simulink model "adip_least_square_MN_sim"  (R2013a)
settings: Solver=ode1  StartTime=0.0  StopTime=max(t)  FixedStep=0.001  RelTol=1e-3
values from neighbouring files (symbols this model uses):
  alpha3 = m2*L1*l2    (= 0.00424944)    [p1c332_adip_id_least_square.m]
  alpha5 = m2*l2*g    (= 0.1836432)    [p1c332_adip_id_least_square.m]
  Tf1 = 0.075    [p1c322_cdip_id_least_square.m]    (also in p1c322_cdip_plot_MN.m = 0.05; p1c332_adip_id_least_square.m)
  Tf2 = 0.075    [p1c322_cdip_id_least_square.m]    (also in p1c322_cdip_plot_MN.m = 0.05; p1c332_adip_id_least_square.m)
libraries: cstblocks x6
settings Model: Creator=kawata  LastModifiedBy=kawata

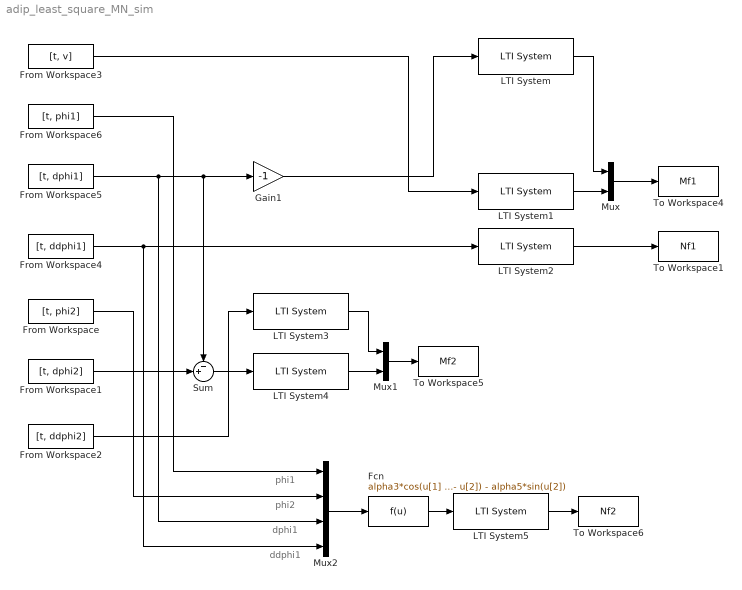
== system adip_least_square_MN_sim ==
  note: phi1
  note: phi2
  note: dphi1
  note: ddphi1
  Fcn : Fcn  Expr=alpha3*cos(u[1] - u[2])*u[4] - alpha3*u[3]^2*sin(u[1] - u[2]) - alpha5*sin(u[2])
  From Workspace : FromWorkspace  VariableName=[t, phi2]  SampleTime=0
  From Workspace1 : FromWorkspace  VariableName=[t, dphi2]  SampleTime=0
  From Workspace2 : FromWorkspace  VariableName=[t, ddphi2]  SampleTime=0
  From Workspace3 : FromWorkspace  VariableName=[t, v]  SampleTime=0
  From Workspace4 : FromWorkspace  VariableName=[t, ddphi1]  SampleTime=0
  From Workspace5 : FromWorkspace  VariableName=[t, dphi1]  SampleTime=0
  From Workspace6 : FromWorkspace  VariableName=[t, phi1]  SampleTime=0
  Gain1 : Gain  Gain=-1  SaturateOnIntegerOverflow=on  OutDataTypeStr=Inherit: Same as input  ParamDataTypeStr=Inherit: Same as input
  LTI System : cstblocks/LTI System  sys=tf(1,[Tf1 1])^3  IC=[]
  LTI System1 : cstblocks/LTI System  sys=tf(1,[Tf1 1])^3  IC=[]
  LTI System2 : cstblocks/LTI System  sys=tf(1,[Tf1 1])^3  IC=[]
  LTI System3 : cstblocks/LTI System  sys=tf(1,[Tf2 1])^3  IC=[]
  LTI System4 : cstblocks/LTI System  sys=tf(1,[Tf2 1])^3  IC=[]
  LTI System5 : cstblocks/LTI System  sys=tf(1,[Tf2 1])^3  IC=[]
  Mux : Mux  Inputs=2
  Mux1 : Mux  Inputs=2
  Mux2 : Mux
  Sum : Sum  Inputs=-+|  SaturateOnIntegerOverflow=on  InputSameDT=on  OutDataTypeStr=Inherit: Same as first input
  To Workspace1 : ToWorkspace  VariableName=Nf1  SampleTime=-1
  To Workspace4 : ToWorkspace  VariableName=Mf1  SampleTime=-1
  To Workspace5 : ToWorkspace  VariableName=Mf2  SampleTime=-1
  To Workspace6 : ToWorkspace  VariableName=Nf2  SampleTime=-1
  wires:
  Mux1/1 -> To Workspace5/1
  LTI System3/1 -> Mux1/1
  LTI System4/1 -> Mux1/2
  From Workspace2/1 -> LTI System3/1
  Mux2/1 -> Fcn/1
  Fcn/1 -> LTI System5/1
  LTI System5/1 -> To Workspace6/1
  From Workspace4/1 -> Mux2/4, LTI System2/1
  Mux/1 -> To Workspace4/1
  LTI System/1 -> Mux/1
  LTI System1/1 -> Mux/2
  LTI System2/1 -> To Workspace1/1
  From Workspace5/1 -> Mux2/3, Sum/1, Gain1/1
  Gain1/1 -> LTI System/1
  From Workspace3/1 -> LTI System1/1
  From Workspace1/1 -> Sum/2
  Sum/1 -> LTI System4/1
  From Workspace/1 -> Mux2/2
  From Workspace6/1 -> Mux2/1
